simulink model "EV_Tractive_Effort_Model"  (R2026a)
settings: Solver=VariableStepAuto

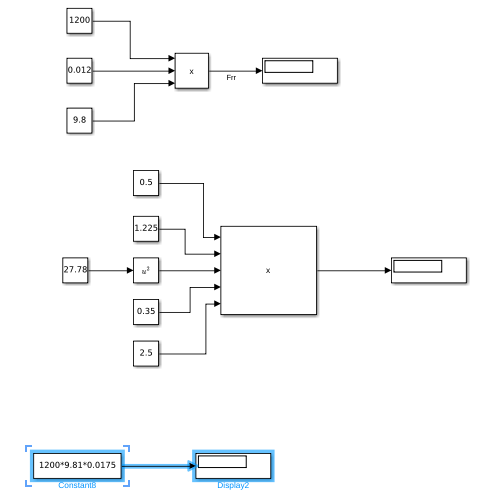
[thumbnail: Simulink's stored preview of the top-level diagram]
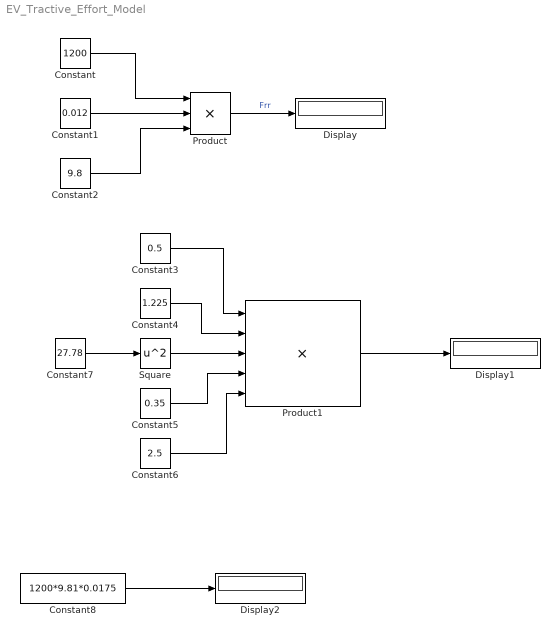
== system EV_Tractive_Effort_Model ==
  Constant : Constant  Value=1200
  Constant1 : Constant  Value=0.012
  Constant2 : Constant  Value=9.8
  Constant3 : Constant  Value=0.5
  Constant4 : Constant  Value=1.225
  Constant5 : Constant  Value=0.35
  Constant6 : Constant  Value=2.5
  Constant7 : Constant  Value=27.78
  Constant8 : Constant  Value=1200*9.81*0.0175
  Display : Display
  Display1 : Display
  Display2 : Display
  Product : Product  Inputs=3
  Product1 : Product  Inputs=5
  Square : Math  Operator=square
  wires:
  Constant/1 -> Product/1
  Constant1/1 -> Product/2
  Constant2/1 -> Product/3
  Product/1 -> Display/1  "Frr"
  Constant7/1 -> Square/1
  Square/1 -> Product1/3
  Constant4/1 -> Product1/2
  Constant3/1 -> Product1/1
  Constant5/1 -> Product1/4
  Constant6/1 -> Product1/5
  Product1/1 -> Display1/1
  Constant8/1 -> Display2/1
